simulink model "pdescen_1819_circulo_PoliformaT"  (R2015b)
settings: Solver=ode4  SolverMode=SingleTasking  StartTime=0.0  StopTime=30  FixedStep=0.02  RelTol=1e-3
undefined symbols (not defined in the file or in its folder): b, kmp, r
settings Model: Creator=avalera  LastModifiedBy=avalera
settings DataIOCC: SaveFormat=Array  SignalLoggingSaveFormat=ModelDataLogs
settings OptimizationCC: ExpressionDepthLimit=2147483647  InitFltsAndDblsToZero=on
settings DebuggingCC: SaveWithParameterizedLinksMsg=none  UnderspecifiedInitializationDetection=Classic  MergeDetectMultiDrivingBlocksExec=none  SignalResolutionControl=TryResolveAllWithWarning  SolverPrmCheckMsg=warning  FcnCallInpInsideContextMsg=EnableAllAsWarning  AllowSymbolicDim=on  StateNameClashWarn=warning
settings HardwareCC: ProdBitPerPointer=32  ProdLargestAtomicFloat=None  ProdIntDivRoundTo=Undefined  ProdEndianess=Unspecified  ProdWordSize=32  ProdHWDeviceType=32-bit Generic
settings GRTTargetCC: TargetFcnLib=ansi_tfl_tmw.mat  GeneratePreprocessorConditionals=Disable all  CombineOutputUpdateFcns=off  GRTInterface=on
settings ConfigComp: CovModelRefEnable=Off

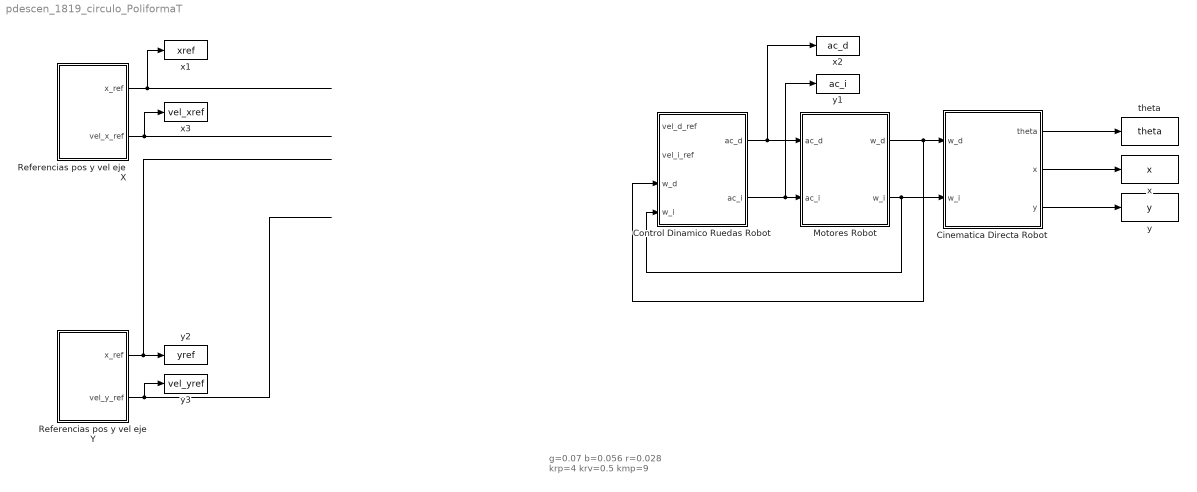
== system pdescen_1819_circulo_PoliformaT ==
  note: g=0.07
      | b=0.056
      | r=0.028
      | krp=4
      | krv=0.5
      | kmp=9
  Cinematica Directa Robot : Subsystem
  Control Dinamico Ruedas Robot : Subsystem
  Motores Robot : Subsystem
  Referencias pos y vel eje Y : Subsystem
  Referencias pos y vel eje X : Subsystem
  theta : ToWorkspace  VariableName=theta  SampleTime=-1
  x : ToWorkspace  VariableName=x  SampleTime=-1
  x1 : ToWorkspace  VariableName=xref  SampleTime=-1
  x2 : ToWorkspace  VariableName=ac_d  SampleTime=-1
  x3 : ToWorkspace  VariableName=vel_xref  SampleTime=-1
  y : ToWorkspace  VariableName=y  SampleTime=-1
  y1 : ToWorkspace  VariableName=ac_i  SampleTime=-1
  y2 : ToWorkspace  VariableName=yref  SampleTime=-1
  y3 : ToWorkspace  VariableName=vel_yref  SampleTime=-1
  wires:
  Cinematica Directa Robot/1(theta) -> theta/1
  Cinematica Directa Robot/3(y) -> y/1
  Referencias pos y vel eje X/2(vel_x_ref) -> x3/1
  Referencias pos y vel eje X/1(x_ref) -> x1/1
  Referencias pos y vel eje Y/1(x_ref) -> y2/1
  Referencias pos y vel eje Y/2(vel_y_ref) -> y3/1
  Cinematica Directa Robot/2(x) -> x/1
  Control Dinamico Ruedas Robot/1(ac_d) -> x2/1, Motores Robot/1(ac_d)
  Control Dinamico Ruedas Robot/2(ac_i) -> y1/1, Motores Robot/2(ac_i)
  Motores Robot/2(w_i) -> Cinematica Directa Robot/2(w_i), Control Dinamico Ruedas Robot/4(w_i)
  ? -> Control Dinamico Ruedas Robot/1(vel_d_ref)
  ? -> Control Dinamico Ruedas Robot/2(vel_i_ref)
  Motores Robot/1(w_d) -> Control Dinamico Ruedas Robot/3(w_d), Cinematica Directa Robot/1(w_d)

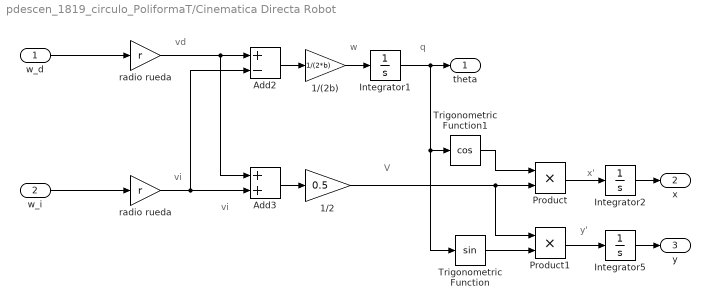
== system pdescen_1819_circulo_PoliformaT/Cinematica Directa Robot ==
  note: vi
  note: x'
  note: y'
  note: vd
  note: V
  note: q
  note: w
  note: vi
  w_d : Inport
  w_i : Inport  Port=2
  1/(2b) : Gain  Gain=1/(2*b)
  1/2 : Gain  Gain=0.5
  Add2 : Sum  Inputs=+-
  Add3 : Sum
  Integrator1 : Integrator
  Integrator2 : Integrator  InitialCondition=0.35
  Integrator5 : Integrator
  Product : Product  RndMeth=Zero
  Product1 : Product  RndMeth=Zero
  Trigonometric Function : Trigonometry
  Trigonometric Function1 : Trigonometry  Operator=cos
  radio rueda : Gain  Gain=r
  "radio rueda " : Gain  Gain=r
  theta : Outport
  x : Outport  Port=2
  y : Outport  Port=3
  wires:
  radio rueda/1 -> Add2/1, Add3/1
  "radio rueda "/1 -> Add3/2, Add2/2
  Integrator5/1 -> y/1
  Trigonometric Function/1 -> Product1/2
  1/(2b)/1 -> Integrator1/1
  Add3/1 -> 1/2/1
  1/2/1 -> Product1/1, Product/2
  Add2/1 -> 1/(2b)/1
  Integrator1/1 -> theta/1, Trigonometric Function1/1, Trigonometric Function/1
  Trigonometric Function1/1 -> Product/1
  Product/1 -> Integrator2/1
  w_i/1 -> "radio rueda "/1
  w_d/1 -> radio rueda/1
  Integrator2/1 -> x/1
  Product1/1 -> Integrator5/1

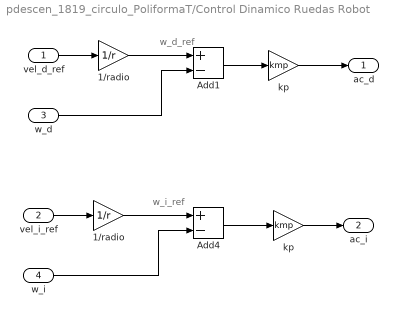
== system pdescen_1819_circulo_PoliformaT/Control Dinamico Ruedas Robot ==
  note: w_i_ref
  note: w_d_ref
  vel_d_ref : Inport
  vel_i_ref : Inport  Port=2
  w_d : Inport  Port=3
  w_i : Inport  Port=4
  1/radio : Gain  Gain=1/r
  "1/radio " : Gain  Gain=1/r
  Add1 : Sum  Inputs=+-
  Add4 : Sum  Inputs=+-
  kp : Gain  Gain=kmp
  "kp " : Gain  Gain=kmp
  ac_d : Outport
  ac_i : Outport  Port=2
  wires:
  vel_i_ref/1 -> "1/radio "/1
  vel_d_ref/1 -> 1/radio/1
  Add4/1 -> "kp "/1
  Add1/1 -> kp/1
  1/radio/1 -> Add1/1
  "1/radio "/1 -> Add4/1
  w_d/1 -> Add1/2
  w_i/1 -> Add4/2
  kp/1 -> ac_d/1
  "kp "/1 -> ac_i/1

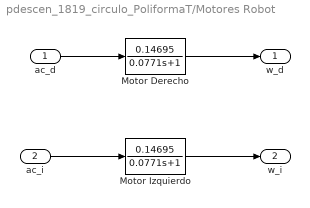
== system pdescen_1819_circulo_PoliformaT/Motores Robot ==
  ac_d : Inport
  ac_i : Inport  Port=2
  Motor Derecho : TransferFcn  Numerator=[0.14695]  Denominator=[0.0771 1]
  Motor Izquierdo : TransferFcn  Numerator=[0.14695]  Denominator=[0.0771 1]
  w_d : Outport
  w_i : Outport  Port=2
  wires:
  ac_i/1 -> Motor Izquierdo/1
  ac_d/1 -> Motor Derecho/1
  Motor Izquierdo/1 -> w_i/1
  Motor Derecho/1 -> w_d/1

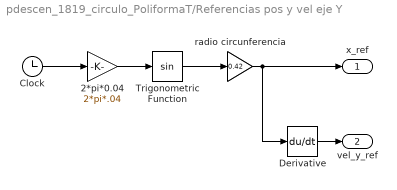
== system pdescen_1819_circulo_PoliformaT/Referencias pos y vel eje Y ==
  2*pi*0.04 : Gain  Gain=2*pi*.04  SampleTime=0.02
  Clock : Clock
  Derivative : Derivative
  Trigonometric Function : Trigonometry
  radio circunferencia : Gain  Gain=0.42
  x_ref : Outport
  vel_y_ref : Outport  Port=2
  wires:
  Derivative/1 -> vel_y_ref/1
  radio circunferencia/1 -> x_ref/1, Derivative/1
  Clock/1 -> 2*pi*0.04/1
  2*pi*0.04/1 -> Trigonometric Function/1
  Trigonometric Function/1 -> radio circunferencia/1

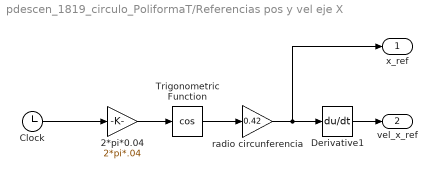
== system pdescen_1819_circulo_PoliformaT/Referencias pos y vel eje X ==
  2*pi*0.04 : Gain  Gain=2*pi*.04  SampleTime=0.02
  Clock : Clock
  Derivative1 : Derivative
  Trigonometric Function : Trigonometry  Operator=cos
  radio circunferencia : Gain  Gain=0.42
  x_ref : Outport
  vel_x_ref : Outport  Port=2
  wires:
  Derivative1/1 -> vel_x_ref/1
  radio circunferencia/1 -> x_ref/1, Derivative1/1
  Clock/1 -> 2*pi*0.04/1
  2*pi*0.04/1 -> Trigonometric Function/1
  Trigonometric Function/1 -> radio circunferencia/1
